simulink model "PR_3_var2"  (R2020b)
settings: Solver=VariableStepAuto  StartTime=0.0  StopTime=0.005  FixedStep=1e-4  RelTol=1e-3
undefined symbols (not defined in the file): Ja, Ke, Km, La, Ms, Ra
libraries: simulink x4
settings Model: Creator=SIA  LastModifiedBy=SIA

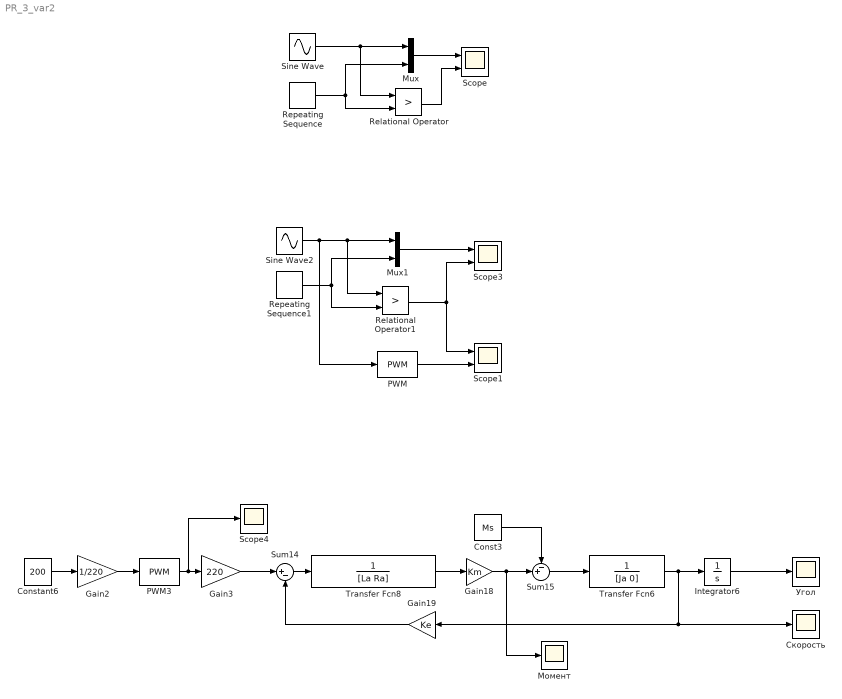
== system PR_3_var2 ==
  Const3 : Constant  Value=Ms
  Constant6 : Constant  Value=200
  Gain18 : Gain  Gain=Km
  Gain19 : Gain  Gain=Ke
  Gain2 : Gain  Gain=1/220
  Gain3 : Gain  Gain=220
  Integrator6 : Integrator
  Mux : Mux  Inputs=2
  Mux1 : Mux  Inputs=2
  PWM : simulink/Discontinuities/PWM  DisableCoverage=on  Period=0.2  DisallowZeroDutyCycle=off  RunAtFixedTimeIntervals=on  SampleTime=0.001
  PWM3 : simulink/Discontinuities/PWM  DisableCoverage=on  Period=5e-5  DisallowZeroDutyCycle=off  RunAtFixedTimeIntervals=on  SampleTime=0.0000001
  Relational Operator : RelationalOperator  Operator=>  OutDataTypeStr=boolean  RndMeth=Simplest
  Relational Operator1 : RelationalOperator  Operator=>  OutDataTypeStr=boolean  RndMeth=Simplest
  Repeating Sequence : simulink/Sources/Repeating Sequence  rep_seq_t=[0 0.1]  rep_seq_y=[0 1]
  Repeating Sequence1 : simulink/Sources/Repeating Sequence  rep_seq_t=[0 0.2]  rep_seq_y=[0 1]
  Scope : Scope  NumInputPorts=2
  Scope1 : Scope  NumInputPorts=2
  Scope3 : Scope  NumInputPorts=2
  Scope4 : Scope
  Sine Wave : Sin  SampleTime=0
  Sine Wave2 : Sin  SampleTime=0
  Sum14 : Sum  Inputs=|+-
  Sum15 : Sum  Inputs=-+|
  Transfer Fcn6 : TransferFcn  Denominator=[Ja 0]
  Transfer Fcn8 : TransferFcn  Denominator=[La Ra]
  Момент : Scope
  Скорость : Scope
  Угол : Scope
  wires:
  Relational Operator/1 -> Scope/2
  Mux/1 -> Scope/1
  Sine Wave/1 -> Relational Operator/1, Mux/1
  Repeating Sequence/1 -> Relational Operator/2, Mux/2
  Sine Wave2/1 -> PWM/1, Relational Operator1/1, Mux1/1
  Mux1/1 -> Scope3/1
  Repeating Sequence1/1 -> Relational Operator1/2, Mux1/2
  Relational Operator1/1 -> Scope1/1, Scope3/2
  PWM/1 -> Scope1/2
  Integrator6/1 -> Угол/1
  Const3/1 -> Sum15/1
  Transfer Fcn8/1 -> Gain18/1
  Gain19/1 -> Sum14/2
  Transfer Fcn6/1 -> Скорость/1, Gain19/1, Integrator6/1
  Gain18/1 -> Момент/1, Sum15/2
  Sum14/1 -> Transfer Fcn8/1
  Sum15/1 -> Transfer Fcn6/1
  PWM3/1 -> Scope4/1, Gain3/1
  Constant6/1 -> Gain2/1
  Gain2/1 -> PWM3/1
  Gain3/1 -> Sum14/1
